simulink model "NumSim_standard_eVTOL"  (R2024b)
settings: Solver=ode14x  StartTime=0.0  StopTime=250  FixedStep=0.005  RelTol=1e-3
values from neighbouring files (symbols this model uses):
  aDl =     [initdata.mat]
  aDr =     [initdata.mat]
  aDyn =     [initdata.mat]
  Airport = init_airport('PHNL')    [initdata_HIL_eVTOL.m]
  aLat =     [initdata.mat]
  aLon =     [initdata.mat]
  D = Prop.D    [EOM_dt_MC.m]    (also in EOM_get_alf_dt_de_prop_evtol.m = CD * QS)
  dt0 = X(2)    [EOM_get_alf_dt_de_prop_evtol.m]    (also in initdata.mat = 0.258252593971; initdata_HIL_eVTOL.m = EOM_dt_MC)
  EAS0 = TAS0 / EAS2TAS    [initdata_HIL_eVTOL.m]
  FCS = init_FCS    [initdata_HIL_eVTOL.m]
  General = init_layoutdata    [EOM_dt_MC.m]    (also in build_optimized_CA.m; initdata.mat = ; initdata_HIL_eVTOL.m)
  h0 = Con(1)    [EOM_get_alf_dt_de_prop_evtol.m]    (also in initdata.mat = 450; initdata_HIL_eVTOL.m = 50)
  mass = Con(3)    [EOM_get_alf_dt_de_prop_evtol.m]    (also in initdata.mat = 2255.54; initdata_HIL_eVTOL.m = 7)
  Motor = init_motor_evtol    [EOM_dt_MC.m]    (also in initdata.mat = []; initdata_HIL_eVTOL.m)
  Prop = init_propeller_evtol_new    [EOM_dt_MC.m]    (also in initdata_HIL_eVTOL.m)
  R2D = 180/pi    (= 57.2957795131)    [EOM_get_alf_dt_de_prop_evtol.m]    (also in init_FCS.m; init_aerodata_evtol.m; init_airport.m; initdata.mat)
  theta0 = -0.0510981441662    [initdata.mat]
undefined symbols (not defined in the file or in its folder): A1, aDa, aDe, asbhl20env, B1, C1, de0, Earth, Environment, InitData, Kd, Kp, magnitude, Tc, WGS84
libraries: simulink_extras x26, simulink x18, slpidlib x14, vrlib x8, matrix_library x6, sharedutil x6, sharedtransform x5, aerolibwindfilters x4, aerolibatmos2 x3, aerolibobsolete x2, aerolibactuator x2, aerolibasang x2
(part 7 of 7)

== stateflow chart NumSim_standard_eVTOL/FCS/FCS CMD/Mode Generator ==
  note: LonMod:
      | 1-theta hold
      | 2-height hold
      | 3-gamma control
      | 4-landing flare control
      | 5-TakeOff
      |
      | LatMod:
      | 1-phi hold
      | 2-lateral deviation control
      | 3-taxi y control
  note: FlightMod
      | 1-Ready
      | 2-TakeOff
      | 3-PullUp
      | 4-Climb
      | 5-Cruise, 5.1-circle, 5.2-line
      | 6-Return
      | 7-Approach
      | 8-Flare
      | 9-TouchDown
      | 10-Taxi
      | 11-GoAround
      | 12-Parachute
  state Pull1 [commented out]
    entry:FlightMod=4;
    Lonmod=1;
    thetac=-5/57.3;
    Vmod=1;
    Vc=14;
    Latmod=1;
    phic=0;
    L1mod=2;
  state cruise
    entry:FlightMod=5;
    %Lonmod=3;
    gammac=0/57.3;
    Lonmod=2;
    hc=50;
    thetac=0/57.3;
    Vmod=4;
    Vc=13;
    Latmod=2;
    phic=0;
    L1mod=2;
    chic=0;
    yc=0;
  state Climb
    entry:FlightMod=4;
    Lonmod=2;
    %gammac=15/57.3;
    %Lonmod=2;
    hc=50;
    Vmod=4;
    Vc=22.76;
    Latmod=1;
    phic=0;
    L1mod=2;
    icmd=0
  state Glide_Gamma [commented out]
    entry:FlightMod=6;
    Lonmod=2;
    hc=h0-0.5757*(time);
    %gammac=-3/57.3;
    Vmod=4;
    Vc=11.1;
    Latmod=2;
    chic=0;
    yc=0;
    L1mod=2;
  note: VMod:
      | 1-cruise throt
      | 2-max throt
      | 3-min throt
      | 4-TECS
      | 5-Flare dt Fade
  state Pull
    entry:FlightMod=3;
    Lonmod=1;
    thetac=2/57.3;
    Vmod=4;
    hc=50;
    Vc=22.76;
    Latmod=1;
    phic=0;
    L1mod=2;
    icmd=0;
  state Pull2
    entry:FlightMod=6;
    Lonmod=1;
    thetac=2/57.3;
    Vmod=4;
    %hc=50;
    Vc=2;
    Latmod=1;
    phic=0;
    L1mod=2;
    icmd=1.57;
  state TakeOff
    entry:FlightMod=2;
    Lonmod=5;
    thetac=0/57.3;
    gammac=0/57.3;
    Vmod=2;
    hc=h0+49;
    Vc = 0;
    Latmod=3
    phic=0/57.3;
    chic=0;
    L1mod=2;
    yc=0;
    icmd=1.57;
  state Trim_hc [commented out]
    entry:FlightMod=5;
    Lonmod=1;
    thetac=-90/57.3;
    hc=h0+10;
    Vmod=1;
    Vc=EAS0;
    Latmod=1;
    phic=0/57.3;
    L1mod=2;
    yc=0;
  state Trim_thetac [commented out]
    entry:FlightMod=5;
    Lonmod=2;
    thetac=0;
    hc=h0+0;
    Vmod=4;
    Vc=EAS0;
    Latmod=1;
    phic=0/57.3;
    L1mod=2;
    yc=0;
  state Return [commented out]
    entry:FlightMod=6;
    %Lonmod=3;
    %gammac=-3/57.3;
    Lonmod=2;
    hc=h0+0;
    Vmod=4;
    Vc=EAS0;
    Latmod=2;
    phic=0;
    L1mod=2;
  state TakeOn
    entry:FlightMod=7;
    Lonmod=4;
    thetac=0/57.3;
    gammac=0/57.3;
    Vmod=5;
    hc=h0+1;
    Vc = 2;
    Latmod=3
    phic=0/57.3;
    chic=0;
    L1mod=2;
    yc=0;
    icmd=1.57;
  cruise -> ? [commented out] : [LAND_SW==1]
  Climb -> cruise : [H>=48&&time>=100]
  Pull1 -> ? [commented out] : [time>=7]
  Pull -> Climb : [V>=21 ]
  Glide_Gamma -> ? [commented out] : [H<=h_runway+8]
  cruise -> Pull2 : [V<=14&&time>140]
  TakeOff -> Pull : [H>=49  && time>=30]
  Trim_hc -> ? [commented out] : [time>=0]
  Pull2 -> TakeOn : [V<=8]
  (default) -> TakeOff
  Return -> ? [commented out] : [H<=h_runway+5.4]
  data: FlightMod output; H input; x input; V input; h_runway input; Lonmod output; thetac output; gammac output; hc output; Vmod output; Vc output; Latmod output; phic output; chic output; yc output double; time input; L1mod output; EAS0 parameter; h0 parameter; i local; psi0 input; LAND_SW input; icmd output

== matlab function NumSim_standard_eVTOL/FCS/MATLAB Function1 ==
  data: u input; y output
function y = fcn(u)
y=0;
if u<=3 || u>=6
    y=1;
end

== matlab function NumSim_standard_eVTOL/FCS/MATLAB Function2 ==
  data: u input; y output
function y = fcn(u)
y=0;
if u>=3 && u<=6
    y=1;
end

== matlab function NumSim_standard_eVTOL/FCS/MC/Pxy control/MATLAB Function ==
  data: a_x input; phi_c output; a_y input; psi input; g input; theta_c output
function [phi_c, theta_c] = fcn(a_x,a_y,psi,g)
%a_x,a_y是经过速度环pid控制之后的输出
%yaw是实际的yaw角度,单位是弧度制,并且matlab的三角函数接收的是弧度制
%g是重力加速度
%输出的角度也是弧度制

A_INV = [ sin(psi)  -cos(psi);
          cos(psi)  sin(psi)];

desire_phi_theta = -1*(1/g) * A_INV * [a_x;a_y]; 

phi_c = desire_phi_theta(1);
theta_c = desire_phi_theta(2);

if desire_phi_theta(1) > pi/18
    phi_c = pi/18;
elseif desire_phi_theta(1) < -pi/18
    phi_c = -pi/18;
end

if desire_phi_theta(2) > pi/18
    theta_c = pi/18;
elseif desire_phi_theta(2) < -pi/18
    theta_c = -pi/18;
end

== matlab function NumSim_standard_eVTOL/FCS/MATLAB Function ==
  data: FlightMod input; dl_cmd output; da_MC input; de_MC input; dr_MC input; dt_MC input; i input; pos_plr input; de_FW input; dr_FW input; da_FW input; dt_FW input; Va input; dr_cmd output; da_cmd output; dt_final output
function [dl_cmd, dr_cmd, da_cmd, dt_final] = Transition_Mixer(FlightMod, da_MC, de_MC, dr_MC, dt_MC,  i, pos_plr, de_FW, dr_FW, da_FW, dt_FW, Va)

    dt_final = zeros(6,1);
    dl_cmd = 0.0; dr_cmd = 0.0; da_cmd = 0.0;
    
    lim_rad = 25 * pi / 180;

    %权重计算
    V_start = 3; 
    V_end   = 22.76; 
    
    if Va <= V_start
        gamma_aero = 0.0;%气动舵面权重
    elseif Va >= V_end
        gamma_aero = 1.0;
    else
        %gamma_aero = 0.5 * (1 - cos(pi * (Va - V_start) / (V_end - V_start)));
        gamma_aero=(Va-V_start)/19.76;
    end

    if Va <= 18.0
        gamma_thrust = 0.0;%油门权重
    elseif Va >= 22.76
        gamma_thrust = 1.0;
    else
        %gamma_thrust = 0.5 * (1 - cos(pi * (Va - 55.0) / 10.0));
        gamma_thrust =(Va-18)/4.76;
    end

    %权重约束
    if FlightMod <= 2 || FlightMod >=6
        gamma_aero = 0.0;
        gamma_thrust = 0.0;
    elseif FlightMod == 3
        gamma_aero = gamma_aero;
        gamma_thrust = gamma_thrust; 
    else
        gamma_aero = 1.0;
        gamma_thrust = 1.0;
    end

    %动力指令解算预处理
    dt0_hover = [0.509; 0.505; 0.501; 0.501; 0.505;0.509]; %旋翼配平油门
    dt0_FW    = 0.554; % 固定翼巡航配平油门

    MC_roll_dem   = da_MC *(1 - gamma_aero);
    MC_pitch_dem  = de_MC *(1 - gamma_aero);
    MC_yaw_dem    = dr_MC *(1 - gamma_aero);
    MC_thrust_dem = dt_MC *1;%(1 - gamma_thrust);

   
    %控制分配和输出逻辑
  
    if FlightMod <= 2 || FlightMod >=6
        %悬停
        delta_dt = get_Dynamic_Allocation(MC_roll_dem, MC_pitch_dem, MC_yaw_dem, MC_thrust_dem, pos_plr, i);
        dt_final = delta_dt + dt0_hover;
        
        dl_cmd = 0.0;
        dr_cmd = 0.0;
        da_cmd = 0.0;

    elseif FlightMod == 3
        %过渡
        delta_dt = get_Dynamic_Allocation(MC_roll_dem, MC_pitch_dem, MC_yaw_dem, MC_thrust_dem, pos_plr, i);
        
  
        %dt_final = gamma_thrust * ((dt_FW + dt0_FW) * ones(6, 1)) + (1 - gamma_thrust) * (delta_dt + dt0_hover);
        %
        %dt_final = (1 - gamma_aero) * dt0_hover + gamma_aero * (dt_FW + dt0_FW) + delta_dt;
        %dt_final=sin(i)*(delta_dt + dt0_hover)+cos(i)*((dt_FW + dt0_FW) * ones(6, 1));

        dt_final=(1-gamma_thrust)*(delta_dt + dt0_hover)+gamma_thrust*((dt_FW + dt0_FW) * ones(6, 1));

        % 气动舵面渐入与V尾解耦
        dl_cmd = gamma_aero * (de_FW - dr_FW);
        dr_cmd = gamma_aero * (dr_FW + de_FW);
        da_cmd = gamma_aero * da_FW;

    elseif FlightMod >= 4
        % 爬升＋巡航
        dt_final = (dt_FW + dt0_FW) * ones(6, 1);
        
        dl_cmd = de_FW - dr_FW;
        dr_cmd = dr_FW + de_FW;
        da_cmd = da_FW;
    end
 
    %限幅
    dl_cmd = max(-lim_rad, min(lim_rad, dl_cmd));
    dr_cmd = max(-lim_rad, min(lim_rad, dr_cmd));
    da_cmd = max(-lim_rad, min(lim_rad, da_cmd));

    for k = 1:6
        dt_final(k) = max(0.0, min(1.0, dt_final(k))); 
    end
end

function dt = get_Dynamic_Allocation(da_MC, de_MC, dr_MC, dt_MC, pos_plr, i)

    L1_x = pos_plr(1);  L1_y = pos_plr(2);
    L2_x = pos_plr(4);  L2_y = pos_plr(5);
    L3_x = pos_plr(7);  L3_y = pos_plr(8);
    L4_x = pos_plr(10); L4_y = pos_plr(11);
    L5_x = pos_plr(13); L5_y = pos_plr(14);
    L6_x = pos_plr(16); L6_y = pos_plr(17);
    
    positions_x = [L1_x, L2_x, L3_x, L4_x, L5_x, L6_x];
    positions_y = [L1_y, L2_y, L3_y, L4_y, L5_y, L6_y];
    max_position = max([abs(positions_x), abs(positions_y)]);
    
    %设定最小值防止奇异点
    eff_i = max(i, 0.1); 
    sin_i = sin(eff_i);
    cos_i = cos(eff_i);
    
    %映射
     C_thrust = [1/0.509, 1/0.505, 1/0.501, 1/0.501, 1/0.505, 1/0.509]; 
    C_roll   = -positions_y / max_position;                    
    C_pitch  = positions_x / max_position;                     
    C_yaw_Q  = [-1, 1, 1, -1, -1, 1]; 
    
    CA_dyn = zeros(4, 6);
    CA_dyn(1, :) = C_thrust; 
    CA_dyn(2, :) = C_roll * sin_i;
    CA_dyn(3, :) = C_pitch * sin_i;
    
    K_diff = 1.0; 
    CA_dyn(4, :) = (C_yaw_Q * sin_i) + (C_roll * cos_i * K_diff);
    
    %求伪逆分配
    lambda = 1e-4;
    CA_pinv = CA_dyn' / (CA_dyn * CA_dyn' + lambda * eye(4));
    
    act_MC = [dt_MC; da_MC; de_MC; dr_MC];
    dt0 = CA_pinv * act_MC;
    
    % 6. 输出
    dt = zeros(6,1);
    for k = 1:6
        dt(k,1) = dt0(k);
    end
end
